simulink model "fig913_cont"  (R2017a)
settings: Solver=FixedStepAuto  StartTime=0.0  StopTime=runtime  FixedStep=dt  RelTol=1e-3  EnableMultiTasking=on
values from neighbouring files (symbols this model uses):
  e = 5    [test_round.m]    (also in test_straight.m = 10)
settings Model: Creator=a01209720  LastModifiedBy=a01209720
settings SolverCC: AutoInsertRateTranBlk=on
settings DataIOCC: LimitDataPoints=on
settings OptimizationCC: LifeSpan=inf
settings DebuggingCC: AllowSymbolicDim=off  SFUnexpectedBacktrackingDiag=warning  SFNoUnconditionalDefaultTransitionDiag=warning  SFExecutionAtInitializationDiag=none
settings GRTTargetCC: TargetLangStandard=C89/C90 (ANSI)
settings ConfigComp: CovMetricSettings=dw  CovHtmlReporting=on  CovSaveCumulativeToWorkspaceVar=on  CovSaveSingleToWorkspaceVar=on  CovShowResultsExplorer=off  CovExternalEMLEnable=off

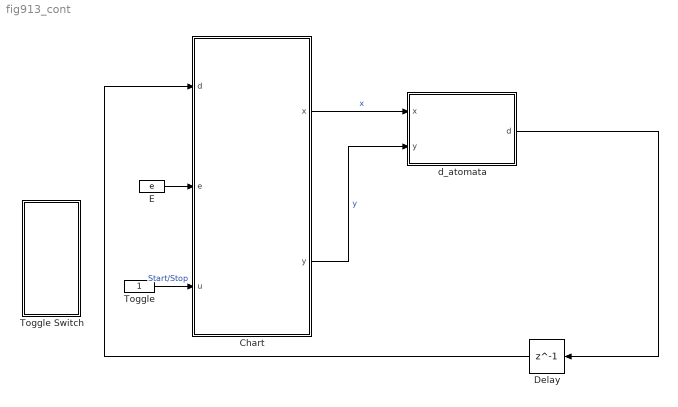
== system fig913_cont ==
  Chart : Stateflow chart  TreatAsAtomicUnit=on
  Delay : Delay  DelayLength=1  InitialCondition=0
  E : Constant  Value=e
  Toggle : Constant
  Toggle Switch : Subsystem  DialogController=hmiCreateDDGDialog  IsWebBlock=on  mask(MWDashboardBlock){webBlockId=9ce7b99b-8eaf-4cd0-9f7a-8e2d2923029e, webBlockType=toggleswitch, ShowInLibBrowser=on, ShowInitialText=on, HMISrcModelName=fig913_cont}
      mask prompts: webBlockId "WebBlock Id"; webBlockType "WebBlock Type"; HMISrcModelName "Source Model"
      mask help: SimulinkHMI:dialogs:SwitchDialogDesc
      mask Help: helpview([docroot '/mapfiles/simulink.map'], 'hmi_toggle_switch')
      mask Display:
      | if strcmp(get_param(bdroot(gcb),'BlockDiagramType'), 'library')
      |     image([(matlabroot) '/toolbox/simulink/hmi/icons/ToggleSwitch.png']);
      | end
  d_atomata : MATLAB Function  TreatAsAtomicUnit=on
  wires:
  E/1 -> Chart/2(e)
  Chart/1(x) -> d_atomata/1(x)  "x"
  Toggle/1 -> Chart/3(u)  "Start/Stop"
  Chart/2(y) -> d_atomata/2(y)  "y"
  d_atomata/1(d) -> Delay/1
  Delay/1 -> Chart/1(d)

== system fig913_cont/Toggle Switch ==

== matlab function fig913_cont/d_atomata ==
  data: x input; d output; y input
function d = fcn(x,y)
  d = sqrt(x^2+y^2)- 46.0977;
  assert(1.5*5>d>-1.5*5);

== stateflow chart fig913_cont/Chart ==
  settings: updateMethod=CONTINUOUS
  state Right %State Name
    du:
    x_dot = ((v*cos(dir))/2); % entry action
    y_dot = ((v*sin(dir))/2); % entry action
    dir_dot =- pi;
    %d >= e
    % during:
  state Straight
    du:
    x_dot = (v*cos(dir)); % entry action
    y_dot = (v*sin(dir)); % entry action
    dir_dot = 0;
    %-e <= d <= e
  state Stop
    du: x_dot = 0; %x0;
    y_dot = 0; %y0;
    dir_dot = 0; %theta0;
  state Left
    du:
    x_dot = ((v*cos(dir))/2); % entry action
    y_dot = ((v*sin(dir))/2); % entry action
    dir_dot=pi;
  Right %State Name -> Straight [order 1] : [d <= e]
      | % [transition condition]{action}
  Straight -> Right %State Name [order 1] : [d >= e]
  Straight -> Left [order 3] : [d <= -e]
  Left -> Straight [order 1] : [d >= -e]
  Straight -> Stop [order 2] : [u == 0]
  Stop -> Straight [order 2] : [u == 1 & -e <= d <= e]
  Right %State Name -> Stop [order 2] : [u == 0]
  Stop -> Right %State Name [order 1] : [u == 1 & d >= e]
  (default) -> Stop
  Left -> Stop [order 2] : [u == 0]
  Stop -> Left [order 3] : [u == 1 & d <= -e]
  Stop -> Stop [order 4]
  data: x output =x0; y output =y0; d input; e input; u input; dir local double =theta0; v constant double =v; dt constant double =dt
  data x settings: updateMethod=SF_CONTINUOUS_TIME_DATA
  data y settings: updateMethod=SF_CONTINUOUS_TIME_DATA
  data dir settings: updateMethod=SF_CONTINUOUS_TIME_DATA
